simulink model "BlinkLED"  (R2016a)
settings: Solver=FixedStepAuto  StartTime=0.0  StopTime=inf  RelTol=1e-3
libraries: simulink x1
settings Model: Creator=Usuario  LastModifiedBy=willi
settings DataIOCC: LimitDataPoints=on  SaveFormat=Array
settings OptimizationCC: DefaultParameterBehavior=Inlined  OptimizeModelRefInitCode=on  LifeSpan=Inf
settings HardwareCC: ProdBitPerPointer=32  ProdLargestAtomicFloat=None  ProdIntDivRoundTo=Undefined  ProdEndianess=Unspecified  ProdWordSize=32  ProdHWDeviceType=32-bit Generic
settings ModelReferenceCC: PropagateSignalLabelsOutOfModel=off
settings RTWCC: SystemTargetFile=ert.tlc  TemplateMakefile=ert_default_tmf  GenerateReport=on  CustomInclude=Interface.h  IncludeHyperlinkInReport=on  LaunchReport=on  GenerateTraceInfo=on  GenerateTraceReport=on  GenerateTraceReportSl=on  GenerateTraceReportSf=on  GenerateTraceReportEml=on
settings CodeAppCC: ForceParamTrailComments=on  IgnoreCustomStorageClasses=off  OperatorAnnotations=on  SimulinkDataObjDesc=on  SFDataObjDesc=on  MATLABFcnDesc=on  InsertBlockDesc=on  MATLABSourceComments=on
settings ERTTargetCC: InlinedParameterPlacement=NonHierarchical  ERTCustomFileTemplate=example_file_process.tlc
settings ConfigComp: CovModelRefEnable=Off

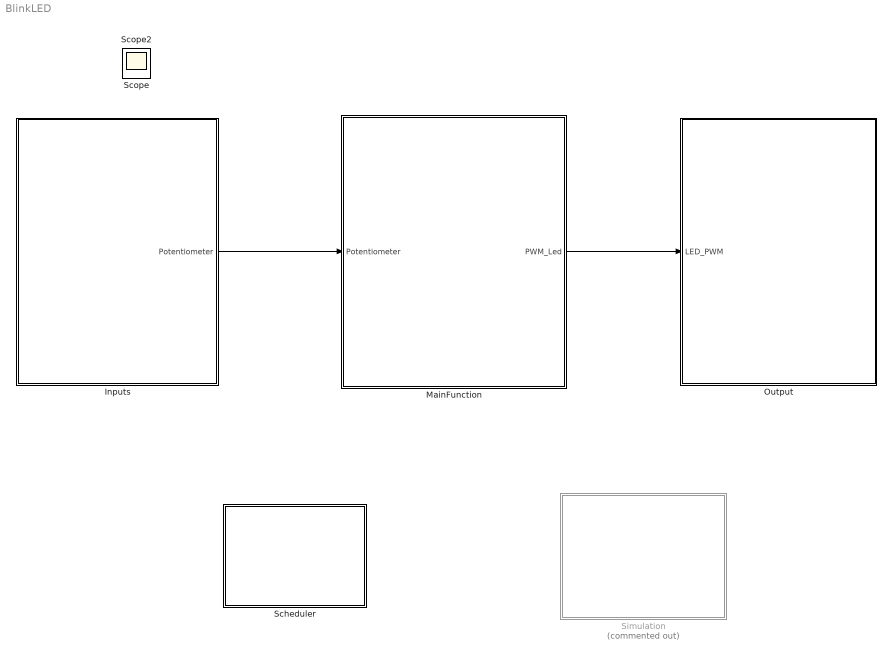
== system BlinkLED ==
  Inputs : Subsystem
  MainFunction : Subsystem
  Output : Subsystem
  Scheduler : Subsystem
  Simulation : Subsystem  Commented=on
  Scope : Scope
  Scope2 : Scope
  wires:
  MainFunction/1(PWM_Led) -> Output/1(LED_PWM)
  Inputs/1(Potentiometer) -> MainFunction/1(Potentiometer)

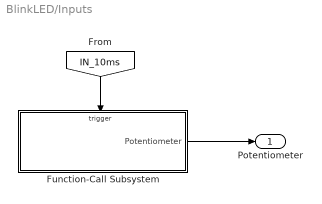
== system BlinkLED/Inputs ==
  Function-Call Subsystem : Subsystem  TreatAsAtomicUnit=on
  Potentiometer : Outport
  wires:
  [IN_10ms] -> Function-Call Subsystem/Trigger
  Function-Call Subsystem/1(Potentiometer) -> Potentiometer/1

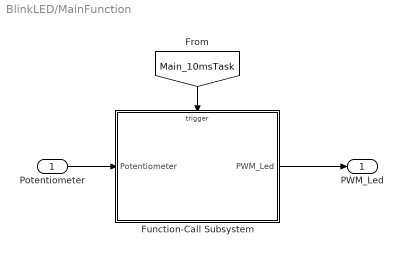
== system BlinkLED/MainFunction ==
  Potentiometer : Inport
  Function-Call Subsystem : Subsystem  TreatAsAtomicUnit=on
  PWM_Led : Outport
  wires:
  [Main_10msTask] -> Function-Call Subsystem/Trigger
  Function-Call Subsystem/1(PWM_Led) -> PWM_Led/1
  Potentiometer/1 -> Function-Call Subsystem/1(Potentiometer)

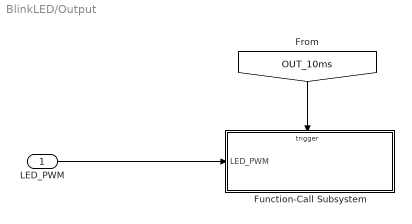
== system BlinkLED/Output ==
  LED_PWM : Inport
  Function-Call Subsystem : Subsystem  TreatAsAtomicUnit=on
  wires:
  LED_PWM/1 -> Function-Call Subsystem/1(LED_PWM)
  [OUT_10ms] -> Function-Call Subsystem/Trigger

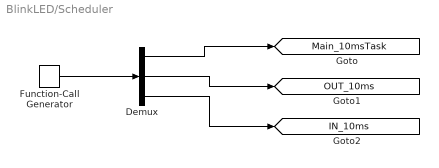
== system BlinkLED/Scheduler ==
  Demux : Demux  Outputs=3
  Function-Call Generator : simulink/Ports & Subsystems/Function-Call Generator  sample_time=0.01  numberOfIterations=1
  tag scope: IN_10ms=global, Main_10msTask=global, OUT_10ms=global
  wires:
  Function-Call Generator/1 -> Demux/1
  Demux/1 -> [Main_10msTask]
  Demux/2 -> [OUT_10ms]
  Demux/3 -> [IN_10ms]

== system BlinkLED/Simulation ==

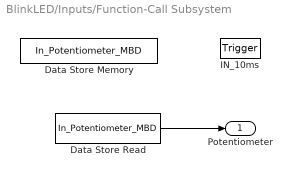
== system BlinkLED/Inputs/Function-Call Subsystem ==
  IN_10ms : TriggerPort  TriggerType=function-call  VariantControl=Variant
  Data Store Memory : DataStoreMemory  DataStoreName=In_Potentiometer_MBD  ReadBeforeWriteMsg=warning  WriteAfterWriteMsg=warning  WriteAfterReadMsg=warning  ShowAdditionalParam=off  OutDataTypeStr=uint32
  Data Store Read : DataStoreRead  DataStoreName=In_Potentiometer_MBD
  Potentiometer : Outport
  wires:
  Data Store Read/1 -> Potentiometer/1

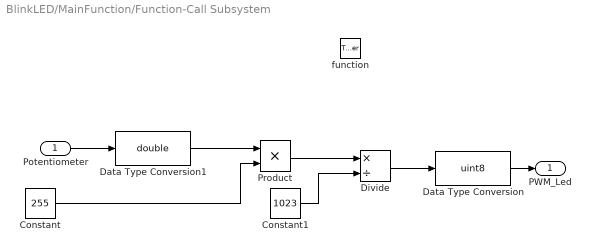
== system BlinkLED/MainFunction/Function-Call Subsystem ==
  Potentiometer : Inport
  function : TriggerPort  TriggerType=function-call  VariantControl=Variant
  Constant : Constant  Value=255
  Constant1 : Constant  Value=1023
  Data Type Conversion : DataTypeConversion  OutDataTypeStr=uint8
  Data Type Conversion1 : DataTypeConversion  OutDataTypeStr=double
  Divide : Product  Inputs=*/  OutDataTypeStr=double
  Product : Product  OutDataTypeStr=double
  PWM_Led : Outport
  wires:
  Potentiometer/1 -> Data Type Conversion1/1
  Constant/1 -> Product/2
  Product/1 -> Divide/1
  Constant1/1 -> Divide/2
  Divide/1 -> Data Type Conversion/1
  Data Type Conversion/1 -> PWM_Led/1
  Data Type Conversion1/1 -> Product/1

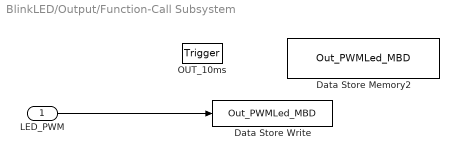
== system BlinkLED/Output/Function-Call Subsystem ==
  LED_PWM : Inport
  OUT_10ms : TriggerPort  TriggerType=function-call  VariantControl=Variant
  Data Store Memory2 : DataStoreMemory  DataStoreName=Out_PWMLed_MBD  ReadBeforeWriteMsg=warning  WriteAfterWriteMsg=warning  WriteAfterReadMsg=warning  ShowAdditionalParam=off  OutDataTypeStr=uint8
  Data Store Write : DataStoreWrite  DataStoreName=Out_PWMLed_MBD
  wires:
  LED_PWM/1 -> Data Store Write/1
